simulink model "without_bias"  (R2019a)
settings: Solver=FixedStepAuto  StartTime=0.0  StopTime=20  FixedStep=0.001  RelTol=1e-3
settings Model: Creator=huic  LastModifiedBy=huic

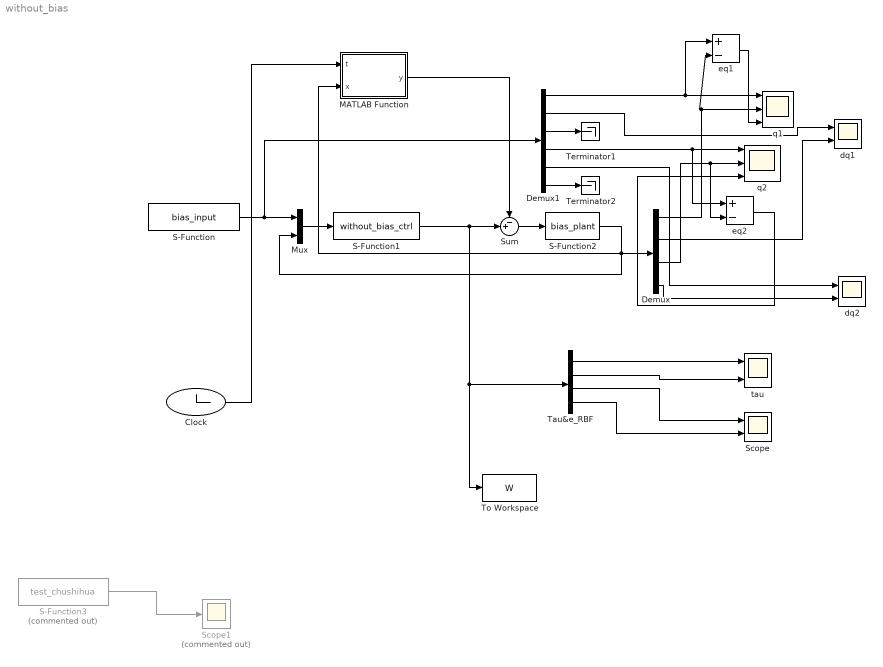
== system without_bias ==
  Clock : Clock
  Demux : Demux
  Demux1 : Demux  Outputs=6
  MATLAB Function : MATLAB Function  TreatAsAtomicUnit=on
  Mux : Mux  Inputs=2
  S-Function : S-Function  FunctionName=bias_input  SFunctionDeploymentMode=off  EnableBusSupport=off
  S-Function1 : S-Function  FunctionName=without_bias_ctrl  SFunctionDeploymentMode=off  EnableBusSupport=off
  S-Function2 : S-Function  FunctionName=bias_plant  SFunctionDeploymentMode=off  EnableBusSupport=off
  S-Function3 : S-Function  Commented=on  FunctionName=test_chushihua  SFunctionDeploymentMode=off  EnableBusSupport=off
  Scope : Scope  NumInputPorts=2
  Scope1 : Scope  Commented=on
  Sum : Sum  Inputs=-+|
  Tau&e_RBF : Demux
  Terminator1 : Terminator
  Terminator2 : Terminator
  To Workspace : ToWorkspace  VariableName=W  SaveFormat=Structure With Time  SampleTime=-1
  dq1 : Scope  NumInputPorts=2
  dq2 : Scope  NumInputPorts=2
  eq1 : Sum  Inputs=+-
  eq2 : Sum  Inputs=+-
  q1 : Scope  NumInputPorts=3
  q2 : Scope  NumInputPorts=3
  tau : Scope  NumInputPorts=2
  wires:
  S-Function1/1 -> Sum/2, To Workspace/1, Tau&e_RBF/1
  S-Function/1 -> Demux1/1, Mux/1
  S-Function2/1 -> MATLAB Function/2(x), Mux/2, Demux/1
  Mux/1 -> S-Function1/1
  Demux1/1 -> eq1/1, q1/1
  Demux/1 -> q1/2, eq1/2
  Demux1/4 -> eq2/1, q2/1
  Demux/3 -> eq2/2, q2/2
  Demux1/2 -> dq1/1
  Demux/2 -> dq1/2
  Demux1/5 -> dq2/1
  Demux/4 -> dq2/2
  Demux1/3 -> Terminator1/1
  Demux1/6 -> Terminator2/1
  Tau&e_RBF/1 -> tau/1
  Tau&e_RBF/2 -> tau/2
  Tau&e_RBF/3 -> Scope/1
  Tau&e_RBF/4 -> Scope/2
  eq1/1 -> q1/3
  eq2/1 -> q2/3
  Sum/1 -> S-Function2/1
  Clock/1 -> MATLAB Function/1(t)
  MATLAB Function/1(y) -> Sum/1
  S-Function3/1 -> Scope1/1

== matlab function without_bias/MATLAB Function ==
  data: t input; y output; x input
function y = turbulence(t,x)
Td=zeros(4,1);
if t>100
    l1 = 0.35;  %unit is 'm'
    l2 = 0.31;  % li is the length of ith link i
    J=[-l1*sin(x(1))+l2*sin(x(1)+x(3))  -l2*sin(x(1)+x(3));  l1*cos(x(1))+l2*cos(x(1)+x(3))  l2*cos(x(1)+x(3)) ];
    Td(1:2,:)=J'*[0,8]';
end
y=Td;
end
